simulink model "test_ba_xe_2"  (R2021b)
settings: Solver=FixedStepAuto  StartTime=0.0  StopTime=40  FixedStep=0.01  RelTol=1e-3
settings Model: Creator=laptop  LastModifiedBy=SPKT2021
settings DataIOCC: ReturnWorkspaceOutputs=off

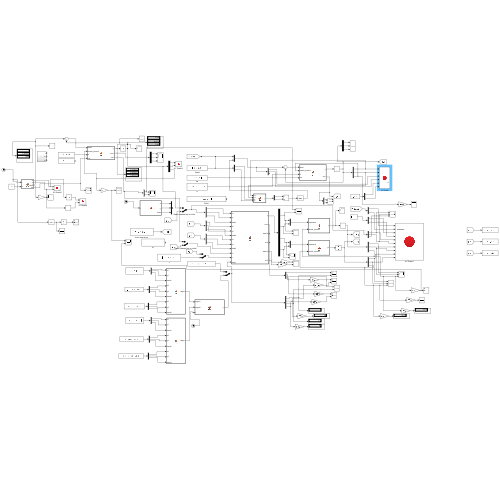
[thumbnail: Simulink's stored preview of the top-level diagram]
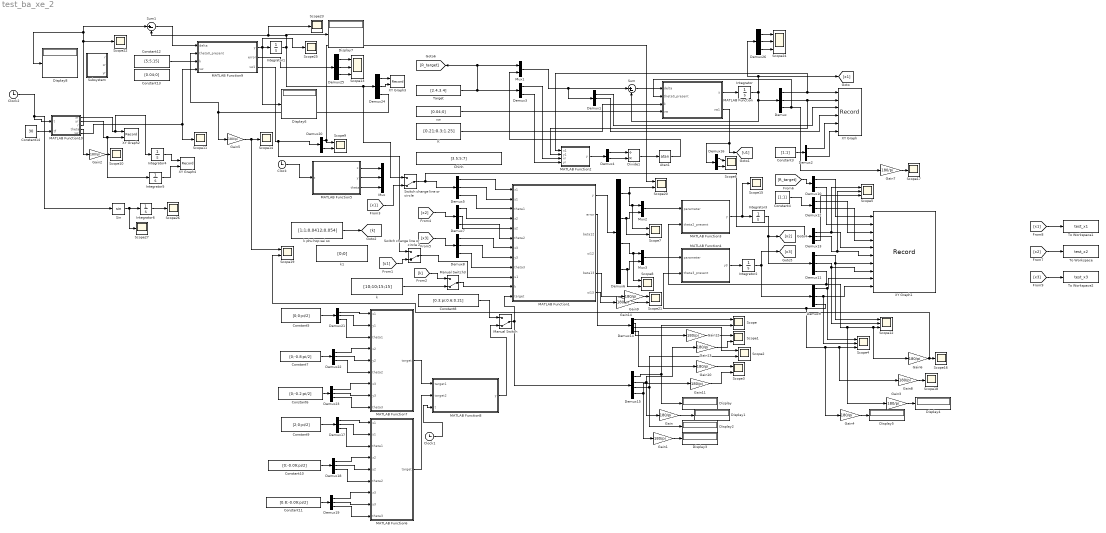
== system test_ba_xe_2 ==
  Atan1 : Trigonometry  Operator=atan
  Chính : Constant  Value=[3.5;5;7]
  Clock : Clock
  Clock1 : Clock
  Clock2 : Clock
  Constant10 : Constant  Value=[0;-0.09;pi/2]
  Constant11 : Constant  Value=[0.8;-0.09;pi/2]
  Constant12 : Constant  Value=[5;5;15]
  Constant13 : Constant  Value=[0.04;0]
  Constant14 : Constant  Value=30
  Constant3 : Constant  Value=[1;1]
  Constant4 : Constant  Value=[1;1]
  Constant5 : Constant  Value=[0;0;pi/2]
  Constant6 : Constant  Value=[0;-0.2;pi/2]
  Constant7 : Constant  Value=[0;-0.8;pi/2]
  Constant8 : Constant  Value=[0.3;pi;0.6;0.21]
  Constant9 : Constant  Value=[2;0;pi/2]
  Demux{,1,5,7..9,11,13,17..19,21..26} (17 alike) : Demux  Outputs=3
  Demux{2..4,10,12,16,20} (7 alike) : Demux  Outputs=2
  Demux14 : Demux
  Demux15 : Demux
  Demux6 : Demux
  Display{,1..8} (9 alike) : Display
  Divide1 : Product  Inputs=/*
  Gain{,1..14} (15 alike) : Gain  Gain=180/pi
  Integrator : Integrator  InitialCondition=[1;1;atan(2.4/1.4)]
  Integrator1 : Integrator  InitialCondition=[3;0;pi/2]
  Integrator2 : Integrator  InitialCondition=[0.8;-0.09;pi/2]
  Integrator3 : Integrator  InitialCondition=[0.1;-0.09;pi/2]
  Integrator4 : Integrator  InitialCondition=[0;0]
  Integrator5 : Integrator  InitialCondition=[0;0]
  Integrator6 : Integrator  InitialCondition=[0;0]
  K : Constant  Value=[0.21;0.3;1.25]
  MATLAB Function : MATLAB Function  TreatAsAtomicUnit=on
  MATLAB Function1 : MATLAB Function  TreatAsAtomicUnit=on
  MATLAB Function10 : MATLAB Function  TreatAsAtomicUnit=on
  MATLAB Function2 : MATLAB Function  TreatAsAtomicUnit=on
  MATLAB Function3 : MATLAB Function  TreatAsAtomicUnit=on
  MATLAB Function4 : MATLAB Function  TreatAsAtomicUnit=on
  MATLAB Function5 : MATLAB Function  TreatAsAtomicUnit=on
  MATLAB Function6 : MATLAB Function  TreatAsAtomicUnit=on
  MATLAB Function7 : MATLAB Function  TreatAsAtomicUnit=on
  MATLAB Function8 : MATLAB Function  TreatAsAtomicUnit=on
  MATLAB Function9 : MATLAB Function  TreatAsAtomicUnit=on
  Manual Switch : ManualSwitch  CurrentSetting=0
  Manual Switch3 : ManualSwitch  CurrentSetting=0
  Mux : Mux  Inputs=3
  Mux1 : Mux  Inputs=2
  Mux2 : Mux  Inputs=2
  Mux3 : Mux  Inputs=2
  Scope{,1..3,6..9,19..21} (11 alike) : Scope  NumInputPorts=2
  Scope{10..11,14..18,22..23,25..27} (12 alike) : Scope
  Scope{4..5,12..13,24} (5 alike) : Scope  NumInputPorts=3
  Sin : Trigonometry
  Subsystem : Subsystem
  Sum : Sum  Inputs=|+-
  Sum1 : Sum  Inputs=|+-
  Switch change line or circle : ManualSwitch  CurrentSetting=0
  Switch change line or circle 2 : ManualSwitch  CurrentSetting=0
  Target : Constant  Value=[2.4,3.4]
  To Workspace : ToWorkspace  VariableName=test_x2  SampleTime=-1
  To Workspace1 : ToWorkspace  VariableName=test_x1  SampleTime=-1
  To Workspace2 : ToWorkspace  VariableName=test_x3  SampleTime=-1
  XY Graph : Record  FileSettingsInternal="{\"entries\":[{\"content\":{\"excelSettings\":{\"content\":{},\"type\":\"Streamout.ExcelSettings\"}},\"type\":\"Streamout.FileSettingStorage\",\"uuid\":\"70fd1e76-0798-47bf-acf1-eed4893097b9\"}],\"packageUris\":[\"http://schema.mathworks.com/mf0/streamout_blocks/R2020a\"],\"version\":\"1.0\"}"  Layout=[1 1]  SignalsInternal="{\"entries\":[{\"content\":{\"signals\":[{\"content\":{\"blockPath\":[\"test_ba_xe_2/XY Graph\"],\"channel\":[],\"dimensions\":[1],\"domain\":\"test_ba_xe_2/XY Graph\",\"lineColor\":\"#a2142f\",\"plots\":[1],\"port\":1,\"sid\":[\"\"],\"signalID\":10247,\"signalName\":\"Demux:1\"},\"type\":\"RecordBlkView.Signal\",\"uuid\":\"22dc617a-e5f8-4a56-a773-12a231c157fd\"},{\"content\":{\"blockPath\":[\"test_ba_xe_2/XY Graph\"],\"channel\":[],\"dimensions\":[1],\"domain\":\"test_ba_xe_2/XY Graph\",\"lineColor\":\"#139fff\",\"plots\":[1],\"port\":2,\"sid\":[\"\"],\"signalID\":10251,\"signalName\":\"Demux:2\"},\"type\":\"RecordBlkView.Signal\",\"uuid\":\"7f2a6346-d4e4-4a26-a5f1-173b5c58d339\"},{\"content\":{\"blockPath\":[\"test_ba_xe_2/XY Graph\"],\"channel\":[],\"dimensions\":[1],\"domain\":\"test_ba_xe_2/XY Graph\",\"lineColor\":\"#0072bd\",\"plots\":[1],\"port\":3,\"sid\":[\"\"],\"signalID\":10305,\"signalName\":\"Demux1:1\"},\"type\":\"RecordBlkView.Signal\",\"uuid\":\"19a52d4f-63f8-4a1c-b345-0646ed3297be\"},{\"content\":{\"blockPath\":[\"test_ba_xe_2/XY Graph\"],\"channel\":[],\"dimensions\":[1],\"domain\":\"test_ba_xe_2/XY Graph\",\"lineColor\":\"#d95319\",\"plots\":[1],\"port\":4,\"sid\":[\"\"],\"signalID\":10309,\"signalName\":\"Demux1:2\"},\"type\":\"RecordBlkView.Signal\",\"uuid\":\"2b4c834e-808f-43f5-a644-199dfab36cd7\"},{\"content\":{\"blockPath\":[\"test_ba_xe_2/XY Graph\"],\"channel\":[],\"dimensions\":[1],\"domain\":\"test_ba_xe_2/XY Graph\",\"lineColor\":\"#edb120\",\"plots\":[],\"port\":5,\"sid\":[\"\"],\"signalID\":10313,\"signalName\":\"Demux2:1\"},\"type\":\"RecordBlkView.Signal\",\"uuid\":\"4960efdb-4bab-41f2-9ba3-19675a5fe83e\"},{\"content\":{\"blockPath\":[\"test_ba_xe_2/XY Graph\"],\"channel\":[],\"dimensions\":[1],\"domain\":\"test_ba_xe_2/XY Graph\",\"lineColor\":\"#7e2f8e\",\"plots\":[],\"port\":6,\"sid\":[\"\"],\"signalID\":10317,\"signalName\":\"Demux2:2\"},\"type\":\"RecordBlkView.Signal\",\"uuid\":\"e0231401-8a03-4c9d-852e-fc1cac34d569\"}]},\"type\":\"RecordBlkView.InputSignals\",\"uuid\":\"ca0fc099-080b-4e9f-9d79-27718017b68b\"}],\"packageUris\":[\"http://schema.mathworks.com/mf0/streamout_blocks/R2020a\"],\"version\":\"1.0\"}"  VisualizationBindings="{\"xyplotplugin\":{\"info\":[{\"series\":[{\"bindingParametersList\":[{\"parameter\":\"X-Axis\",\"signalID\":10247,\"signalName\":\"Demux:1\"},{\"parameter\":\"Y-Axis\",\"signalID\":10251,\"signalName\":\"Demux:2\"}],\"seriesID\":55733},{\"bindingParametersList\":[{\"parameter\":\"X-Axis\",\"signalID\":10305,\"signalName\":\"Demux1:1\"},{\"parameter\":\"Y-Axis\",\"signalID\":10309,\"signalName\":\"Demux1:2\"}],\"seriesID\":7735}],\"subplotID\":1},{\"series\":[],\"subplotID\":2}]}}"  CompatibilityTag=XY
  XY Graph1 : Record  FileSettingsInternal="{\"entries\":[{\"content\":{\"excelSettings\":{\"content\":{},\"type\":\"Streamout.ExcelSettings\"}},\"type\":\"Streamout.FileSettingStorage\",\"uuid\":\"5f21f3b9-ae8d-48b3-8879-12e4856874da\"}],\"packageUris\":[\"http://schema.mathworks.com/mf0/streamout_blocks/R2020a\"],\"version\":\"1.0\"}"  Layout=[1 1]  SignalsInternal="{\"entries\":[{\"content\":{\"signals\":[{\"content\":{\"blockPath\":[\"test_ba_xe_2/XY Graph1\"],\"channel\":[],\"dimensions\":[1,1],\"domain\":\"test_ba_xe_2/XY Graph1\",\"lineColor\":\"#64d413\",\"plots\":[1],\"port\":5,\"sid\":[\"\"],\"signalID\":10255,\"signalName\":\"Demux13:1\"},\"type\":\"RecordBlkView.Signal\",\"uuid\":\"346042b2-c55a-477c-ac58-653c01ef7587\"},{\"content\":{\"blockPath\":[\"test_ba_xe_2/XY Graph1\"],\"channel\":[],\"dimensions\":[1,1],\"domain\":\"test_ba_xe_2/XY Graph1\",\"lineColor\":\"#ff13a6\",\"plots\":[1],\"port\":6,\"sid\":[\"\"],\"signalID\":10259,\"signalName\":\"Demux13:2\"},\"type\":\"RecordBlkView.Signal\",\"uuid\":\"37647398-54f6-4350-83d7-82ee1aaf33a7\"},{\"content\":{\"blockPath\":[\"test_ba_xe_2/XY Graph1\"],\"channel\":[],\"dimensions\":[1,1],\"domain\":\"test_ba_xe_2/XY Graph1\",\"lineColor\":\"#fe330a\",\"plots\":[1],\"port\":7,\"sid\":[\"\"],\"signalID\":10263,\"signalName\":\"Demux11:1\"},\"type\":\"RecordBlkView.Signal\",\"uuid\":\"1d72cf2e-b9af-46d0-ade9-88b83ea02045\"},{\"content\":{\"blockPath\":[\"test_ba_xe_2/XY Graph1\"],\"channel\":[],\"dimensions\":[1,1],\"domain\":\"test_ba_xe_2/XY Graph1\",\"lineColor\":\"#22b573\",\"plots\":[1],\"port\":8,\"sid\":[\"\"],\"signalID\":10267,\"signalName\":\"Demux11:2\"},\"type\":\"RecordBlkView.Signal\",\"uuid\":\"50f5cb63-57c7-409f-b836-57a401cd662e\"},{\"content\":{\"blockPath\":[\"test_ba_xe_2/XY Graph1\"],\"channel\":[],\"dimensions\":[1,1],\"domain\":\"test_ba_xe_2/XY Graph1\",\"lineColor\":\"#a2142f\",\"plots\":[1],\"port\":9,\"sid\":[\"\"],\"signalID\":10271,\"signalName\":\"Demux9:1\"},\"type\":\"RecordBlkView.Signal\",\"uuid\":\"f56de818-f69a-45e8-a192-8a3802260f78\"},{\"content\":{\"blockPath\":[\"test_ba_xe_2/XY Graph1\"],\"channel\":[],\"dimensions\":[1,1],\"domain\":\"test_ba_xe_2/XY Graph1\",\"lineColor\":\"#139fff\",\"plots\":[1],\"port\":10,\"sid\":[\"\"],\"signalID\":10275,\"signalName\":\"Demux9:2\"},\"type\":\"RecordBlkView.Signal\",\"uuid\":\"f5a40c0a-7289-40e2-b054-abd4a4733d62\"},{\"content\":{\"blockPath\":[\"test_ba_xe_2/XY Graph1\"],\"channel\":[],\"dimensions\":[1],\"domain\":\"test_ba_xe_2/XY Graph1\",\"lineColor\":\"#a2142f\",\"plots\":[],\"port\":1,\"sid\":[\"\"],\"signalID\":10321,\"signalName\":\"Demux10:1\"},\"type\":\"RecordBlkView.Signal\",\"uuid\":\"10276834-824d-492b-986e-f61a700b455c\"},{\"content\":{\"blockPath\":[\"test_ba_xe_2/XY Graph1\"],\"channel\":[],\"dimensions\":[1],\"domain\":\"test_ba_xe_2/XY Graph1\",\"lineColor\":\"#139fff\",\"plots\":[],\"port\":2,\"sid\":[\"\"],\"signalID\":10325,\"signalName\":\"Demux10:2\"},\"type\":\"RecordBlkView.Signal\",\"uuid\":\"6ae25923-1dd5-4a47-8d36-005537971680\"},{\"content\":{\"blockPath\":[\"test_ba_xe_2/XY Graph1\"],\"channel\":[],\"dimensions\":[1],\"domain\":\"test_ba_xe_2/XY Graph1\",\"lineColor\":\"#ff6929\",\"plots\":[],\"port\":3,\"sid\":[\"\"],\"signalID\":10329,\"signalName\":\"Demux12:1\"},\"type\":\"RecordBlkView.Signal\",\"uuid\":\"00b5a749-6cba-4e86-8459-4d1a53d686b8\"},{\"content\":{\"blockPath\":[\"test_ba_xe_2/XY Graph1\"],\"channel\":[],\"dimensions\":[1],\"domain\":\"test_ba_xe_2/XY Graph1\",\"lineColor\":\"#b746ff\",\"plots\":[],\"port\":4,\"sid\":[\"\"],\"signalID\":10333,\"signalName\":\"Demux12:2\"},\"type\":\"RecordBlkView.Signal\",\"uuid\":\"95d92f99-1f24-4b84-a753-0123319120b2\"}]},\"type\":\"RecordBlkView.InputSignals\",\"uuid\":\"45551a62-a647-44fe-80ff-8b4d4990277d\"}],\"packageUris\":[\"http://schema.mathworks.com/mf0/streamout_blocks/R2020a\"],\"version\":\"1.0\"}"  VisualizationBindings="{\"xyplotplugin\":{\"info\":[{\"series\":[{\"bindingParametersList\":[{\"parameter\":\"X-Axis\",\"signalID\":10263,\"signalName\":\"Demux11:1\"},{\"parameter\":\"Y-Axis\",\"signalID\":10267,\"signalName\":\"Demux11:2\"}],\"seriesID\":1774},{\"bindingParametersList\":[{\"parameter\":\"Y-Axis\",\"signalID\":10275,\"signalName\":\"Demux9:2\"},{\"parameter\":\"X-Axis\",\"signalID\":10271,\"signalName\":\"Demux9:1\"}],\"seriesID\":41491},{\"bindingParametersList\":[{\"parameter\":\"X-Axis\",\"signalID\":10255,\"signalName\":\"Demux13:1\"},{\"parameter\":\"Y-Axis\",\"signalID\":10259,\"signalName\":\"Demux13:2\"}],\"seriesID\":14095}],\"subplotID\":1},{\"series\":[],\"subplotID\":2},{\"series\":[],\"subplotID\":9},{\"series\":[],\"subplotID\":10}]}}"  CompatibilityTag=XY
  XY Graph2 : Record  FileSettingsInternal="{\"entries\":[{\"content\":{\"excelSettings\":{\"content\":{},\"type\":\"Streamout.ExcelSettings\"}},\"type\":\"Streamout.FileSettingStorage\",\"uuid\":\"ce2218ae-73ce-424a-82e8-631e6707ad33\"}],\"packageUris\":[\"http://schema.mathworks.com/mf0/streamout_blocks/R2020a\"],\"version\":\"1.0\"}"  Layout=[1 1]  SignalsInternal="{\"entries\":[{\"content\":{\"signals\":[{\"content\":{\"blockPath\":[\"test_ba_xe_2/XY Graph2\"],\"channel\":[],\"dimensions\":[1],\"domain\":\"test_ba_xe_2/XY Graph2\",\"lineColor\":\"#0072bd\",\"plots\":[1],\"port\":1,\"sid\":[\"\"],\"signalID\":10279,\"signalName\":\"MATLAB Function10:1\"},\"type\":\"RecordBlkView.Signal\",\"uuid\":\"4fd544fd-dd5f-40e7-a042-fb5d9c48e3c9\"},{\"content\":{\"blockPath\":[\"test_ba_xe_2/XY Graph2\"],\"channel\":[],\"dimensions\":[1],\"domain\":\"test_ba_xe_2/XY Graph2\",\"lineColor\":\"#d95319\",\"plots\":[1],\"port\":2,\"sid\":[\"\"],\"signalID\":10283,\"signalName\":\"MATLAB Function10:2\"},\"type\":\"RecordBlkView.Signal\",\"uuid\":\"168c8faa-c850-4d7b-82a8-4be4bc01ca1f\"}]},\"type\":\"RecordBlkView.InputSignals\",\"uuid\":\"dedef9ed-5bb7-40cd-8b46-14226bb0d2d2\"}],\"packageUris\":[\"http://schema.mathworks.com/mf0/streamout_blocks/R2020a\"],\"version\":\"1.0\"}"  VisualizationBindings="{\"xyplotplugin\":{\"info\":[{\"series\":[{\"bindingParametersList\":[{\"parameter\":\"X-Axis\",\"signalID\":10279,\"signalName\":\"MATLAB Function10:1\"},{\"parameter\":\"Y-Axis\",\"signalID\":10283,\"signalName\":\"MATLAB Function10:2\"}],\"seriesID\":57375}],\"subplotID\":1}]}}"  CompatibilityTag=XY
  XY Graph3 : Record  FileSettingsInternal="{\"entries\":[{\"content\":{\"excelSettings\":{\"content\":{},\"type\":\"Streamout.ExcelSettings\"}},\"type\":\"Streamout.FileSettingStorage\",\"uuid\":\"15e6eb0c-fa5f-4cbc-acf3-3ef9025712ff\"}],\"packageUris\":[\"http://schema.mathworks.com/mf0/streamout_blocks/R2020a\"],\"version\":\"1.0\"}"  Layout=[1 1]  SignalsInternal="{\"entries\":[{\"content\":{\"signals\":[{\"content\":{\"blockPath\":[\"test_ba_xe_2/XY Graph3\"],\"channel\":[],\"dimensions\":[1,1],\"domain\":\"test_ba_xe_2/XY Graph3\",\"lineColor\":\"#0072bd\",\"plots\":[1],\"port\":1,\"sid\":[\"\"],\"signalID\":10287,\"signalName\":\"Demux24:1\"},\"type\":\"RecordBlkView.Signal\",\"uuid\":\"1d0d9f62-fcb1-4517-bbd3-519d39e8a613\"},{\"content\":{\"blockPath\":[\"test_ba_xe_2/XY Graph3\"],\"channel\":[],\"dimensions\":[1,1],\"domain\":\"test_ba_xe_2/XY Graph3\",\"lineColor\":\"#d95319\",\"plots\":[1],\"port\":2,\"sid\":[\"\"],\"signalID\":10291,\"signalName\":\"Demux24:2\"},\"type\":\"RecordBlkView.Signal\",\"uuid\":\"a7d50201-4d24-4043-8124-0d7dfcc332aa\"}]},\"type\":\"RecordBlkView.InputSignals\",\"uuid\":\"e7e15523-658b-4a33-aa5c-e3a711e32e0a\"}],\"packageUris\":[\"http://schema.mathworks.com/mf0/streamout_blocks/R2020a\"],\"version\":\"1.0\"}"  VisualizationBindings="{\"xyplotplugin\":{\"info\":[{\"series\":[{\"bindingParametersList\":[{\"parameter\":\"X-Axis\",\"signalID\":10287,\"signalName\":\"Demux24:1\"},{\"parameter\":\"Y-Axis\",\"signalID\":10291,\"signalName\":\"Demux24:2\"}],\"seriesID\":50301}],\"subplotID\":1}]}}"  CompatibilityTag=XY
  XY Graph4 : Record  FileSettingsInternal="{\"entries\":[{\"content\":{\"excelSettings\":{\"content\":{},\"type\":\"Streamout.ExcelSettings\"}},\"type\":\"Streamout.FileSettingStorage\",\"uuid\":\"44dc336b-df7a-494e-a918-443b50120dff\"}],\"packageUris\":[\"http://schema.mathworks.com/mf0/streamout_blocks/R2020a\"],\"version\":\"1.0\"}"  Layout=[1 1]  SignalsInternal="{\"entries\":[{\"content\":{\"signals\":[{\"content\":{\"blockPath\":[\"test_ba_xe_2/XY Graph4\"],\"channel\":[],\"dimensions\":[2],\"domain\":\"test_ba_xe_2/XY Graph4\",\"hasChildren\":true,\"lineColor\":\"#a2142f\",\"plots\":[],\"port\":1,\"sid\":[\"\"],\"signalID\":10295,\"signalName\":\"Integrator4\"},\"type\":\"RecordBlkView.Signal\",\"uuid\":\"7fee5173-5970-4381-a9be-8d21b6e5e72f\"},{\"content\":{\"blockPath\":[\"test_ba_xe_2/XY Graph4\"],\"channel\":[1],\"dimensions\":[2],\"domain\":\"test_ba_xe_2/XY Graph4\",\"lineColor\":\"#ff13a6\",\"parentID\":10295,\"plots\":[1],\"port\":1,\"sid\":[\"\"],\"signalID\":10296,\"signalName\":\"Integrator4\"},\"type\":\"RecordBlkView.Signal\",\"uuid\":\"53e60ac6-8e54-41f7-9866-24184eb6acb8\"},{\"content\":{\"blockPath\":[\"test_ba_xe_2/XY Graph4\"],\"channel\":[],\"dimensions\":[2],\"domain\":\"test_ba_xe_2/XY Graph4\",\"hasChildren\":true,\"lineColor\":\"#ff6929\",\"plots\":[],\"port\":2,\"sid\":[\"\"],\"signalID\":10300,\"signalName\":\"Integrator5\"},\"type\":\"RecordBlkView.Signal\",\"uuid\":\"4000003b-b562-407e-9a37-7d04c0db62bc\"},{\"content\":{\"blockPath\":[\"test_ba_xe_2/XY Graph4\"],\"channel\":[1],\"dimensions\":[2],\"domain\":\"test_ba_xe_2/XY Graph4\",\"lineColor\":\"#22b573\",\"parentID\":10300,\"plots\":[],\"port\":2,\"sid\":[\"\"],\"signalID\":10301,\"signalName\":\"Integrator5\"},\"type\":\"RecordBlkView.Signal\",\"uuid\":\"62b31be2-7d0c-459a-85a2-05f9a5484e0e\"},{\"content\":{\"blockPath\":[\"test_ba_xe_2/XY Graph4\"],\"channel\":[2],\"dimensions\":[2],\"domain\":\"test_ba_xe_2/XY Graph4\",\"lineColor\":\"#ff6929\",\"parentID\":10295,\"plots\":[1],\"port\":1,\"sid\":[\"\"],\"signalID\":10336,\"signalName\":\"Integrator4\"},\"type\":\"RecordBlkView.Signal\",\"uuid\":\"fdf726e7-4e34-49e2-864e-740f6617c113\"},{\"content\":{\"blockPath\":[\"test_ba_xe_2/XY Graph4\"],\"channel\":[2],\"dimensions\":[2],\"domain\":\"test_ba_xe_2/XY Graph4\",\"lineColor\":\"#b746ff\",\"parentID\":10300,\"plots\":[],\"port\":2,\"sid\":[\"\"],\"signalID\":10337,\"signalName\":\"Integrator5\"},\"type\":\"RecordBlkView.Signal\",\"uuid\":\"d11aa5b6-17fe-4975-a8e1-7c689a012770\"}]},\"type\":\"RecordBlkView.InputSignals\",\"uuid\":\"031f8201-f3ad-4fc0-9efc-eb21ff1ad7e9\"}],\"packageUris\":[\"http://schema.mathworks.com/mf0/streamout_blocks/R2020a\"],\"version\":\"1.0\"}"  VisualizationBindings="{\"xyplotplugin\":{\"info\":[{\"series\":[{\"bindingParametersList\":[{\"parameter\":\"X-Axis\",\"signalID\":10296,\"signalName\":\"Integrator4(1)\"},{\"parameter\":\"Y-Axis\",\"signalID\":10336,\"signalName\":\"Integrator4(2)\"}],\"seriesID\":30388}],\"subplotID\":1}]}}"  CompatibilityTag=XY
  k : Constant  Value=[10;10;15;15]
  k phu hop sai so : Constant  Value=[1;1;0.0412;0.054]
  k1 : Constant  Value=[0;0]
  vw : Constant  Value=[0.04;0]
  wires:
  Demux12/2 -> XY Graph1/4
  Demux5/1 -> MATLAB Function1/1(x1)
  Demux/1 -> MATLAB Function2/1(x1), XY Graph/1
  MATLAB Function5/2(y) -> Mux/2
  Gain/1 -> Display1/1
  Demux3/1 -> MATLAB Function2/3(xr)
  Atan1/1 -> Mux1/2
  Demux11/2 -> Scope12/2, XY Graph1/8
  Demux14/3 -> Scope2/1
  Demux7/3 -> MATLAB Function1/6(theta2)
  MATLAB Function2/1(y) -> Demux4/1
  Demux9/1 -> Scope4/1, XY Graph1/9
  MATLAB Function5/3(theta) -> Mux/3
  Demux1/2 -> XY Graph/4
  Clock/1 -> MATLAB Function5/1(t)
  k phu hop sai so/1 -> [k]
  MATLAB Function3/1(y) -> Scope15/1, Integrator3/1
  Divide1/1 -> Atan1/1
  Demux16/2 -> Scope6/2
  Demux8/1 -> MATLAB Function1/7(x3)
  Demux16/1 -> Scope6/1
  Demux21/1 -> MATLAB Function7/1(x1)
  Demux9/2 -> Scope4/2, XY Graph1/10
  Sum/1 -> MATLAB Function/1(delta)
  MATLAB Function5/1(x) -> Mux/1
  Demux/2 -> MATLAB Function2/2(y1), XY Graph/2
  MATLAB Function1/2(error) -> Demux14/1
  Demux3/2 -> MATLAB Function2/4(yr)
  Demux22/2 -> MATLAB Function7/5(y2)
  Mux1/1 -> Sum/1, Demux1/1
  Demux2/2 -> XY Graph/6
  Target/1 -> [R_target], Mux1/1, Demux3/1
  vw/1 -> MATLAB Function/4(vw)
  Demux1/1 -> XY Graph/3
  Demux21/2 -> MATLAB Function7/2(y1)
  Demux10/2 -> XY Graph1/2
  MATLAB Function/1(y) -> Integrator/1
  [x3] -> Demux8/1
  Demux8/2 -> MATLAB Function1/8(y3)
  Demux15/1 -> Scope/2, Display/1
  Demux6/2 -> Scope7/2, Mux2/2
  Demux2/1 -> XY Graph/5
  Demux6/1 -> Scope20/2, Scope7/1, Mux2/1
  Demux10/1 -> XY Graph1/1
  MATLAB Function/2(vw1) -> Demux16/1, [u1]
  Demux13/1 -> Scope5/1, XY Graph1/5
  Demux4/1 -> Divide1/1
  Demux14/2 -> Gain12/1
  Demux11/1 -> Scope12/1, XY Graph1/7
  Demux5/3 -> MATLAB Function1/3(theta1)
  Integrator3/1 -> Demux11/1, [x2]
  Demux14/4 -> Gain10/1
  Demux5/2 -> MATLAB Function1/2(y1)
  [x2] -> Demux7/1
  Demux15/2 -> Gain13/1, Gain/1
  Constant3/1 -> Demux2/1
  Demux8/3 -> MATLAB Function1/9(theta3)
  Demux7/2 -> MATLAB Function1/5(y2)
  Demux7/1 -> MATLAB Function1/4(x2)
  Demux13/2 -> Scope5/2, XY Graph1/6
  [R_target] -> Demux10/1
  Demux23/1 -> MATLAB Function7/7(x3)
  Demux6/4 -> Scope8/2, Mux3/2
  Mux2/1 -> MATLAB Function3/1(parameter)
  Demux15/3 -> Scope2/2, Display2/1
  Constant4/1 -> Demux12/1
  MATLAB Function4/1(y3) -> Integrator2/1
  Demux22/1 -> MATLAB Function7/4(x2)
  Demux4/2 -> Divide1/2
  K/1 -> MATLAB Function/3(k)
  Manual Switch/1 -> MATLAB Function1/12(target), Demux15/1
  Constant8/1 -> Manual Switch/1
  Constant5/1 -> Demux21/1
  Demux15/4 -> Gain11/1, Gain1/1
  MATLAB Function1/1(y) -> Demux6/1
  Integrator2/1 -> [x3], Demux9/1
  Demux23/2 -> MATLAB Function7/8(y3)
  Demux14/1 -> Scope/1
  Demux22/3 -> MATLAB Function7/6(theta2)
  Demux12/1 -> XY Graph1/3
  Integrator/1 -> Sum/2, Demux/1, Demux26/1, [x1]
  Demux21/3 -> MATLAB Function7/3(theta1)
  Demux23/3 -> MATLAB Function7/9(theta3)
  Demux19/3 -> MATLAB Function6/9(theta3)
  Demux17/3 -> MATLAB Function6/3(theta1)
  Demux18/3 -> MATLAB Function6/6(theta2)
  Demux19/2 -> MATLAB Function6/8(y3)
  Constant9/1 -> Demux17/1
  Demux18/1 -> MATLAB Function6/4(x2)
  Constant10/1 -> Demux18/1
  Demux19/1 -> MATLAB Function6/7(x3)
  MATLAB Function6/1(target) -> MATLAB Function8/2(target2)
  Demux17/2 -> MATLAB Function6/2(y1)
  Demux18/2 -> MATLAB Function6/5(y2)
  Demux17/1 -> MATLAB Function6/1(x1)
  Constant11/1 -> Demux19/1
  MATLAB Function7/1(target) -> MATLAB Function8/1(target1)
  MATLAB Function8/1(y) -> Manual Switch/2
  Clock1/1 -> MATLAB Function8/3(t)
  Demux6/3 -> Scope8/1, Mux3/1
  Gain1/1 -> Display3/1
  Constant6/1 -> Demux23/1
  Constant7/1 -> Demux22/1
  Integrator1/1 -> Display7/1, Scope23/1, Sum1/2, Switch change line or circle/1, Demux24/1
  Demux20/2 -> Scope9/2
  MATLAB Function9/3(vw1) -> Switch change line or circle 2/1, Demux20/1
  Demux20/1 -> Scope20/1, Scope9/1
  Gain2/1 -> Scope10/1
  MATLAB Function10/5(vw) -> Scope11/1, MATLAB Function9/4(vw)
  MATLAB Function10/1(xr) -> Integrator4/1, XY Graph2/1
  Constant14/1 -> MATLAB Function10/2(tf)
  Constant12/1 -> MATLAB Function9/3(k)
  MATLAB Function10/4(theta) -> Gain2/1
  Clock2/1 -> Sin/1, MATLAB Function10/1(t)
  MATLAB Function10/2(yr) -> XY Graph2/2, Integrator5/1
  MATLAB Function9/1(y) -> Display6/1, Scope25/1, Integrator1/1
  MATLAB Function10/3(r) -> Scope22/1, Display8/1, Sum1/1
  Sum1/1 -> MATLAB Function9/1(delta)
  Demux13/3 -> Scope5/3
  Switch change line or circle/1 -> Demux13/1, Demux5/1
  [x1] -> Switch change line or circle/2
  Switch change line or circle 2/1 -> MATLAB Function1/10(u1)
  [u1] -> Switch change line or circle 2/2
  Gain3/1 -> Display4/1
  Gain4/1 -> Display5/1
  Manual Switch3/1 -> MATLAB Function1/11(k)
  [k] -> Manual Switch3/1
  k/1 -> Manual Switch3/2
  Demux24/3 -> MATLAB Function9/2(theta0_present), Gain5/1
  Demux25/1 -> Scope13/1
  Demux25/2 -> Scope13/2
  Demux25/3 -> Scope13/3
  MATLAB Function9/2(error) -> Demux25/1
  Demux11/3 -> MATLAB Function3/2(theta2_present), Gain3/1, Gain6/1, Scope12/3
  Gain6/1 -> Scope19/2, Scope16/1
  Gain7/1 -> Scope17/1
  Demux/3 -> Gain7/1, MATLAB Function/2(theta0_present)
  Demux24/1 -> XY Graph3/1
  Demux24/2 -> XY Graph3/2
  Gain8/1 -> Scope18/1
  Demux9/3 -> Gain4/1, Gain8/1, Scope4/3, MATLAB Function4/2(theta3_present)
  Gain10/1 -> Scope3/1
  Gain11/1 -> Scope3/2
  Gain12/1 -> Scope1/1
  Gain13/1 -> Scope1/2
  Gain5/1 -> Scope19/1, Scope14/1
  Gain9/1 -> Scope21/1
  Gain14/1 -> Scope21/2
  Demux26/1 -> Scope24/1
  Demux26/2 -> Scope24/2
  Demux26/3 -> Scope24/3
  MATLAB Function1/6(si13) -> Gain14/1
  MATLAB Function1/5(beta13) -> Gain9/1
  Mux3/1 -> MATLAB Function4/1(parameter)
  Integrator4/1 -> XY Graph4/1
  Integrator5/1 -> XY Graph4/2
  Sin/1 -> Scope27/1, Integrator6/1
  Integrator6/1 -> Scope26/1
  [x2] -> To Workspace/1
  [x1] -> To Workspace1/1
  [x3] -> To Workspace2/1

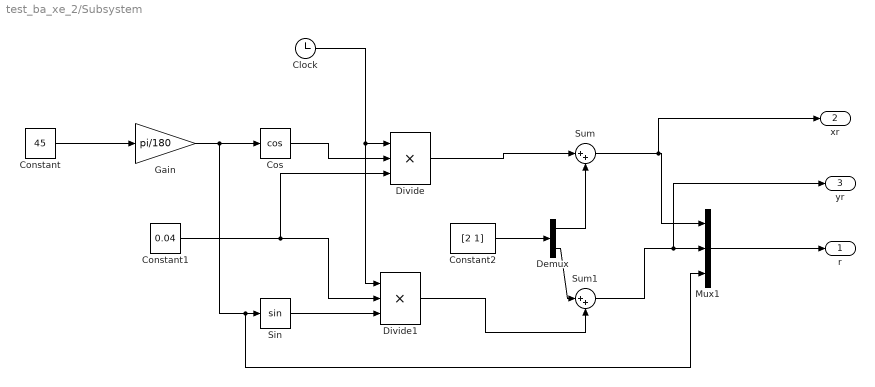
== system test_ba_xe_2/Subsystem ==
  Clock : Clock
  Constant : Constant  Value=45
  Constant1 : Constant  Value=0.04
  Constant2 : Constant  Value=[2 1]
  Cos : Trigonometry  Operator=cos
  Demux : Demux  Outputs=2
  Divide : Product  Inputs=***
  Divide1 : Product  Inputs=***
  Gain : Gain  Gain=pi/180
  Mux1 : Mux  Inputs=3
  Sin : Trigonometry
  Sum : Sum  Inputs=|++
  Sum1 : Sum  Inputs=|++
  r : Outport
  xr : Outport  Port=2
  yr : Outport  Port=3
  wires:
  Cos/1 -> Divide/2
  Demux/2 -> Sum1/1
  Sin/1 -> Divide1/3
  Gain/1 -> Mux1/3, Sin/1, Cos/1
  Sum1/1 -> yr/1, Mux1/2
  Constant/1 -> Gain/1
  Constant1/1 -> Divide1/2, Divide/3
  Clock/1 -> Divide1/1, Divide/1
  Demux/1 -> Sum/2
  Divide/1 -> Sum/1
  Divide1/1 -> Sum1/2
  Sum/1 -> xr/1, Mux1/1
  Constant2/1 -> Demux/1
  Mux1/1 -> r/1

== matlab function test_ba_xe_2/MATLAB Function8 ==
  data: target1 input; y output; target2 input; t input
function y = fcn(target1, target2,t)
% if t<15
%     y = target1;
% else
%     y = target2;
% end
y = target2;

== matlab function test_ba_xe_2/MATLAB Function10 ==
  data: t input; tf input; xr output; yr output; r output; theta output; vw output
function [xr,yr,r,theta,vw] = fcn(t,tf)
radius = 6;
omega = 2*pi/30;
v=omega*radius;

% xr = 5 + 4*cos(theta);
% yr = 5 + 4*sin(theta);

if t<tf
    theta =pi/2+ omega*t;
    xr =  radius*cos(theta - pi/2);
    yr = radius*sin(theta- pi/2);
else
    xr = radius*cos(2*pi);
    yr = radius*sin(2*pi);
    theta =pi/2+ omega*tf;
%     v=0;
%     omega=0;
end
r = [xr;yr;theta];
vw = [v;omega];

== matlab function test_ba_xe_2/MATLAB Function9 ==
  data: delta input; y output; theta0_present input; k input; error output; vw input; vw1 output
function [y,error,vw1]= fcn(delta,theta0_present,k,vw)
A = [cos(theta0_present)   sin(theta0_present) 0;
       -sin(theta0_present) cos(theta0_present) 0;
         0                    0                    1];
e=A*delta;
v=vw(1);
w=vw(2);

V_c=[v*cos(e(3))+k(1)*e(1);
    w + k(2)*v*e(2) + k(3)*v*sin(e(3))];
Matrix = [cos(theta0_present) 0;
          sin(theta0_present) 0;
          0                   1];

% d=0.09;
% Matrix=[cos(theta0_present) -d*sin(theta0_present);
%         sin(theta0_present) d*cos(theta0_present);
%         0                   1];
u=Matrix*V_c;
y = u;
error = e;
vw1 = V_c;

== matlab function test_ba_xe_2/MATLAB Function7 ==
  data: x1 input; target output; y1 input; theta1 input; x2 input; y2 input; theta2 input; x3 input; y3 input; theta3 input
function target = fcn(x1,y1,theta1,x2,y2,theta2,x3,y3,theta3)
%#codegen
d=0.09;
% 
% L12_x=x1-x2-d*cos(theta1);
% L12_y=y1-y2-d*sin(theta1);
% L13_x=x1-x3-d*cos(theta1);
% L13_y=y1-y3-d*sin(theta1);
% L23_x=x2-x3-d*cos(theta2);
% L23_y=y2-y3-d*sin(theta2);
L12_x=x1-x2-d*cos(theta2);
L12_y=y1-y2-d*sin(theta2);
L13_x=x1-x3-d*cos(theta3);
L13_y=y1-y3-d*sin(theta3);
L23_x=x2-x3-d*cos(theta3);
L23_y=y2-y3-d*sin(theta3);

L12=sqrt(L12_x^2+L12_y^2);
L13=sqrt(L13_x^2+L13_y^2);
L23=sqrt(L23_x^2+L23_y^2);

mega12=atan2(L12_y,L12_x)-theta1+pi;
if mega12<0
    k12=fix(-mega12/(2*pi));
    mega12 = 2*(k12+1)*pi +mega12;
end
mega13 = atan2(L13_y,L13_x)-theta1+pi;
if mega13<0 %khi mega <0 se xay ra hien tuong xoay tron
    k13=fix(-mega13/(2*pi));
    mega13 = 2*(k13+1)*pi +mega13;
end
mega23=atan2(L23_y,L23_x)-theta2+pi;
if mega23<0 %khi mega <0 se xay ra hien tuong xoay tron
    k23=fix(-mega23/(2*pi));
    mega23 = 2*(k23+1)*pi +mega23;
end
target=[L12;mega12;L13;mega13];

== matlab function test_ba_xe_2/MATLAB Function1 ==
  data: x1 input; y output; y1 input; theta1 input; x2 input; y2 input; theta2 input; x3 input; y3 input; theta3 input; u1 input; k input; target input; error output; beta12 output; si12 output; beta13 output; si13 output
function [y,error,beta12,si12,beta13,si13] = fcn(x1,y1,theta1,x2,y2,theta2,x3,y3,theta3,u1,k,target)
%#coegen
d=0.09;
% L12_x=x1-x2-d*cos(theta1);
% L12_y=y1-y2-d*sin(theta1);
% L13_x=x1-x3-d*cos(theta1);
% L13_y=y1-y3-d*sin(theta1);
% L23_x=x2-x3-d*cos(theta2);
% L23_y=y2-y3-d*sin(theta2);
L12_x=x1-x2-d*cos(theta2);
L12_y=y1-y2-d*sin(theta2);
L13_x=x1-x3-d*cos(theta3);
L13_y=y1-y3-d*sin(theta3);
L23_x=x2-x3-d*cos(theta3);
L23_y=y2-y3-d*sin(theta3);

L12=sqrt(L12_x^2+L12_y^2);
L13=sqrt(L13_x^2+L13_y^2);
L23=sqrt(L23_x^2+L23_y^2);

mega12=atan2(L12_y,L12_x)-theta1+pi;
if mega12<0
    k12=fix(-mega12/(2*pi));
    mega12 = 2*(k12+1)*pi +mega12;
end
mega13=atan2(L13_y,L13_x)-theta1+pi;
if mega13<0 %khi mega <0 se xay ra hien tuong xoay tron
    k13=fix(-mega13/(2*pi));
    mega13 = 2*(k13+1)*pi +mega13;
end
mega23=atan2(L23_y,L23_x)-theta2+pi;


beta12=theta1-theta2;
beta13=theta1-theta3;
beta23=theta2-theta3;
% if beta12>pi
%     beta12 = pi;
% end
% if beta13>pi
%     beta13 = pi;
% end

si12=beta12+mega12;
si13=beta13+mega13;
si23=beta23+mega23;

% G2=[cos(si12)      d*sin(si12)     0         0;
%     -sin(si12)/L12 d*cos(si12)/L12 0         0;
%     0              0               cos(si13) d*sin(si13);
%     -cos(mega23)   0               cos(si23) d*sin(si23)];
% 
% F2=[-cos(mega12)     0;
%     sin(mega12)/L12 -1;
%     -cos(mega13)     0;
%     0                0];


% p= [k(1)*(target(1)-L12);
%     k(2)*(target(2)-mega12);
%     k(3)*(target(3)-L13);
%     k(4)*(target(4)-L23)];

G12=[cos(si12)      d*sin(si12);
    -sin(si12)/L12 d*cos(si12)/L12;
    ];

F12=[-cos(mega12)     0;
    sin(mega12)/L12  -1];

p12= [k(1)*(target(1)-L12);
    k(2)*(target(2)-mega12)];
%%%%%%
G13=[cos(si13)      d*sin(si13);
    -sin(si13)/L13 d*cos(si13)/L13];

F13=[-cos(mega13)     0;
    sin(mega13)/L13  -1];

p13= [k(1)*(target(3)-L13);
    k(2)*(target(4)-mega13)]; % neu de mega < 0 (-270do =90 do) thi khi tinh
                               %toan cos sin se khong anh huong nhung p3
                               %se bi sai so lon dan den w3 bị vọt lố dao động
% G23=[cos(si23)      d*sin(si23);
%     -sin(si23)/L23 d*cos(si23)/L23];
% 
% F23=[-cos(mega23)     0;
%     sin(mega23)/L23  -1];
% 
% p23= [k(1)*(target(5)-L23);
%     k(2)*(target(6)-mega23)]; % neu de mega < 0 (-270do =90 do) thi khi tinh
%                                %toan cos sin se khong anh huong nhung p3
%                                %se bi sai so lon dan den w3 bị vọt lố dao động
e=[L12;
mega12;
L13;
mega13];


u12=inv(G12)*(p12-F12*u1);
u13=inv(G13)*(p13-F13*u1);
u = [u12(1);u12(2);u13(1);u13(2)];
% u23=inv(G23)*(p23-F23*u1);
% u = [u12(1);u12(2);u23(1);u23(2)];
error=e;
y = u;
% c12=cos(si12)
% s12=sin(si12)
% v12=c12-s12
 
%  %%%%
% x4=1.35;
% y4 =2.0;
% theta4 = 2*pi/3;
% 
% L24_x=x2-x4-d*cos(theta4);
% L24_y=y2-y4-d*sin(theta4);
% 
% L24=sqrt(L24_x^2+L24_y^2);
% sita12 = theta1 - theta2 + mega12;
% sita24 = theta4 - theta2;
% 
% p4 = [k(1)*(target(1) - L12);
%       6*(0.1 - L24)];
% G24 = [cos(sita12) d*sin(sita12);
%        sin(sita24) d*cos(sita24)];
% F4 = [-u1(1)*cos(mega12);0];
% vw4 = inv(G24)*(p4 - F4);
% %%%%%
% 
% %%%%
% x5=2.5;
% y5 =2;
% theta5 = 2*pi/3;
% 
% L35_x=x3-x5-d*cos(theta5);
% L35_y=y3-y5-d*sin(theta5);
% 
% L35=sqrt(L35_x^2+L35_y^2);
% sita13 = theta1 - theta3 + mega13;
% sita35 = theta5 - theta3;
% 
% p5 = [k(1)*(target(3) - L13);
%       5*(0.09 - L35)];
% G35 = [cos(sita13) d*sin(sita13);
%        sin(sita35) d*cos(sita35)];
% F5 = [-u1(1)*cos(mega13);0];
% vw5 = inv(G35)*(p5 - F5);
% %%%%%
% 
% if L24<0.1
%     y = [vw4(1);vw4(2);u(3);u(4)];
% elseif L35 < 0.09
%         y = [u(1);u(2);vw5(1);vw5(2)];
% elseif (L35 < 0.1)&&(L24<0.1)
%         y = [vw4(1);vw4(2);vw5(1);vw5(2)];
% else
%     y=u;
% end

== matlab function test_ba_xe_2/MATLAB Function ==
  data: delta input; y output; theta0_present input; k input; vw input; vw1 output
function [y,vw1] = fcn(delta,theta0_present,k,vw)
%#codegen
A=[cos(theta0_present)   sin(theta0_present) 0;
    -sin(theta0_present) cos(theta0_present) 0;
    0                    0                    1];
e=A*delta;
V_c=[vw(1)*cos(e(3))+k(1)*e(1);
    vw(2)+k(2)*vw(1)*e(2)+k(3)*vw(1)*sin(e(3))];
Matrix=[cos(theta0_present) 0;
        sin(theta0_present) 0;
        0                   1];
u=Matrix*V_c;
y = u;
vw1=V_c;

== matlab function test_ba_xe_2/MATLAB Function2 ==
  data: x1 input; y output; y1 input; xr input; yr input
function y = fcn(x1,y1,xr,yr)
%#codegen
x_delta=xr-x1;
y_delta=yr-y1;
u=[x_delta;y_delta];
y = u;

== matlab function test_ba_xe_2/MATLAB Function3 ==
  data: parameter input; y output; theta2_present input
function y = fcn(parameter,theta2_present)
%#codegen
d=0.09;
Matrix=[cos(theta2_present) -d*sin(theta2_present);
        sin(theta2_present) d*cos(theta2_present);
        0                   1];
% Matrix=[cos(theta2_present) 0;
%         sin(theta2_present) 0;
%         0                   1];
u=Matrix*parameter;
y = u;

== matlab function test_ba_xe_2/MATLAB Function4 ==
  data: parameter input; y3 output; theta3_present input
function y3 = fcn(parameter,theta3_present)
%#codegen
d=0.09;
Matrix=[cos(theta3_present) -d*sin(theta3_present);
        sin(theta3_present) d*cos(theta3_present);
        0                   1];
% Matrix=[cos(theta3_present) 0;
%         sin(theta3_present) 0;
%         0                   1];
u=Matrix*parameter;
y3 = u;

== matlab function test_ba_xe_2/MATLAB Function5 ==
  data: x output; t input; y output; theta output
function [x,y,theta] = fcn(t)
%#codegen
x = (t^3)/1000;
y = t;

theta = pi/2;

== matlab function test_ba_xe_2/MATLAB Function6 ==
  data: x1 input; target output; y1 input; theta1 input; x2 input; y2 input; theta2 input; x3 input; y3 input; theta3 input
function target = fcn(x1,y1,theta1,x2,y2,theta2,x3,y3,theta3)
%#codegen
d=0.09;
% 
% L12_x=x1-x2-d*cos(theta1);
% L12_y=y1-y2-d*sin(theta1);
% L13_x=x1-x3-d*cos(theta1);
% L13_y=y1-y3-d*sin(theta1);
% L23_x=x2-x3-d*cos(theta2);
% L23_y=y2-y3-d*sin(theta2);
L12_x=x1-x2-d*cos(theta2);
L12_y=y1-y2-d*sin(theta2);
L13_x=x1-x3-d*cos(theta3);
L13_y=y1-y3-d*sin(theta3);
L23_x=x2-x3-d*cos(theta3);
L23_y=y2-y3-d*sin(theta3);

L12=sqrt(L12_x^2+L12_y^2);
L13=sqrt(L13_x^2+L13_y^2);
L23=sqrt(L23_x^2+L23_y^2);

mega12=atan2(L12_y,L12_x)-theta1+pi;
if mega12<0
    k12=fix(-mega12/(2*pi));
    mega12 = 2*(k12+1)*pi +mega12;
end
mega13 = atan2(L13_y,L13_x)-theta1+pi;
if mega13<0 %khi mega <0 se xay ra hien tuong xoay tron
    k13=fix(-mega13/(2*pi));
    mega13 = 2*(k13+1)*pi +mega13;
end
% mega23=atan2(L23_y,L23_x)-theta2+pi;
% if mega23<0 %khi mega <0 se xay ra hien tuong xoay tron
%     k23=fix(-mega23/(2*pi));
%     mega23 = 2*(k23+1)*pi +mega23;
% end
target=[L12;mega12;L13;mega13];
